simulink model "soc_dvbs2_fpga"  (R2025b)
settings: Solver=FixedStepDiscrete  StartTime=0.0  StopTime=0  RelTol=1e-3
InitFcn:
  | soc_dvbs2_init;
values from neighbouring files (symbols this model uses):
  Rsym = 4e6    (= 4000000)    [soc_dvbs2_init.m]
  soc_dvbs2_txPacketBits = [1 1 0 1 0 1 1 1 0 1 1 1 ... (2972 elements, 2972x1)]    [soc_dvbs2_txPacketBits.mat]
  syncWord = (dec2bin(hex2dec('AC')) - '0').'    [soc_dvbs2_init.m]
  txDataOut = txobj(frameBits(:))    [soc_dvbs2_init.m]
  txFiltCoeff = txobj.pTxFilterCoeff    [soc_dvbs2_init.m]
undefined symbols (not defined in the file or in its folder): Add, coefficientsLog, coefficientsSqrt1, coefficientsSqrt2, dataBits, designMultirateFIR, noisePow, NumBits1, NumBits2, seedsURNG1, seedsURNG2, Shift, Slope1, Slope2, soc_dvbs2_designFIRFilter, txDataOutS1, txDataOutS10, txDataOutS12, txDataOutS13, txDataOutS14, txDataOutS15, txDataOutS16, txDataOutS18, txDataOutS19, txDataOutS2, txDataOutS20, txDataOutS21, txDataOutS22, txDataOutS24, txDataOutS25, txDataOutS26, txDataOutS27, txDataOutS3, txDataOutS4, txDataOutS5, txDataOutS6, txDataOutS7, txDataOutS8, txDataOutS9
libraries: simulink x214, hdlsllib x211, dspsigops x22, dsphdlfiltering2 x8, dsphdlsigops2 x5, commseqgen3 x5, dsphdlmathfun2 x3, hwlogicconnlib x2, whdledac x2, commhdlcrc x2, whdlutilities x1, whdlmod x1
(part 10 of 12)

== system soc_dvbs2_fpga/DVBS2/DVBS2 TxRx/DVB-S2 HDL Receiver/Synchronizer and PL Header Decoder/Time Frequency and Coarse Phase Synchronizer/Fine Frequency Synchronizer/Modified L and R Algorithm/L and R Algorithm 18 point/Compute R(m) for 13 to 18/Compute R(m)_1 ==
  z : Inport
  zvalid : Inport  Port=2
  Add3 : Sum  Inputs=++|  OutDataTypeStr=Inherit: Inherit via back propagation
  Compare To Constant : simulink/Logic and Bit Operations/Compare To Constant  relop=>=  const=m  OutDataTypeStr=boolean
  Compare To Constant2 : simulink/Logic and Bit Operations/Compare To Constant  relop===  const=N - 1  OutDataTypeStr=boolean
  Complex Multiplier : Subsystem  VariantControl=Use 3 multipliers and 5 adders
      mask Display: disp(['Complex Multiplier' newline 'Latency = 8']);
  Data Type Duplicate : DataTypeDuplicate
  Data Type Conversion : DataTypeConversion  Commented=through  OutDataTypeStr=fixdt(1,28,17)  SaturateOnIntegerOverflow=off  RndMeth=Floor
  Delay : Delay  DelayLength=m
  Delay{1..2,7..9,11..12,14..15} (9 alike) : Delay  DelayLength=1
  Delay{3..6,10,13,16..26} (17 alike) : Delay
  Delay{27..30} (4 alike) : Delay  DelayLength=8
  Gain : Gain  Gain=MulDivFactor  ParamDataTypeStr=Inherit: Inherit from 'Gain'  OutDataTypeStr=Inherit: Same as input
  HDL Counter : hdlsllib/Sources/HDL Counter  CountType=Count limited  CountInit=0  CountStep=1  CountMax=N-1  CountFromType=Initial value  CountFrom=0  CountResetPort=off  CountLoadPort=off  CountEnbPort=on  CountDirPort=off  CountHitOutputPort=off  CountDataType=Unsigned  CountWordLen=nextpow2(N-1)  CountFracLen=0  CountSampTime=1
  Logical Operator : Logic  AllPortsSameDT=off  OutDataTypeStr=boolean
  Logical Operator1 : Logic  AllPortsSameDT=off  OutDataTypeStr=boolean
  Math Function : Math  Operator=conj
  Unit Delay Enabled Synchronous : hdlsllib/Discrete/Unit Delay Enabled Synchronous  InitialCondition=0.0  SampleTime=-1
  Unit Delay Enabled Resettable Synchronous : hdlsllib/Discrete/Unit Delay Enabled Resettable Synchronous  InitialCondition=0.0  SampleTime=-1
  Out1 : Outport
  wires:
  Data Type Conversion/1 -> Delay13/1
  Delay30/1 -> Delay20/1
  Delay29/1 -> Compare To Constant2/1
  Delay28/1 -> Compare To Constant/1
  Delay27/1 -> Delay17/1
  Delay13/1 -> Delay21/1
  Complex Multiplier/1(Out1) -> Data Type Conversion/1
  Delay26/1 -> Delay1/1
  Logical Operator/1 -> Delay25/1
  Delay24/1 -> Unit Delay Enabled Resettable Synchronous/2
  Delay23/1 -> Delay24/1
  Delay22/1 -> Add3/2, Data Type Duplicate/1
  Delay21/1 -> Gain/1
  Gain/1 -> Delay22/1
  Unit Delay Enabled Synchronous/1 -> Out1/1
  Delay20/1 -> Logical Operator/2
  Delay19/1 -> Logical Operator/1
  Delay18/1 -> Logical Operator1/2
  Delay17/1 -> Logical Operator1/1
  Delay16/1 -> Delay30/1
  Delay15/1 -> Delay16/1
  Delay12/1 -> Delay6/1
  Delay11/1 -> Delay5/1
  Delay10/1 -> Delay27/1
  Delay9/1 -> Delay10/1
  Delay8/1 -> Delay4/1
  Delay7/1 -> Delay3/1
  Delay6/1 -> Delay29/1
  Delay5/1 -> Delay28/1
  Delay4/1 -> Complex Multiplier/2(In2)
  Delay3/1 -> Complex Multiplier/1(In1)
  Delay2/1 -> Delay/1, Delay7/1
  Delay14/1 -> HDL Counter/1, Delay15/1, Delay9/1
  Math Function/1 -> Delay8/1
  z/1 -> Delay2/1
  Delay/1 -> Math Function/1
  Delay1/1 -> Unit Delay Enabled Resettable Synchronous/3, Unit Delay Enabled Synchronous/2
  Unit Delay Enabled Resettable Synchronous/1 -> Add3/1, Unit Delay Enabled Synchronous/1
  zvalid/1 -> Delay14/1
  Delay25/1 -> Delay26/1
  Compare To Constant2/1 -> Delay19/1
  Compare To Constant/1 -> Delay18/1
  HDL Counter/1 -> Delay12/1, Delay11/1
  Add3/1 -> Unit Delay Enabled Resettable Synchronous/1, Data Type Duplicate/2
  Logical Operator1/1 -> Delay23/1

== system soc_dvbs2_fpga/DVBS2/DVBS2 TxRx/DVB-S2 HDL Receiver/Synchronizer and PL Header Decoder/Time Frequency and Coarse Phase Synchronizer/Fine Frequency Synchronizer/Modified L and R Algorithm/L and R Algorithm 18 point/Compute R(m) for 13 to 18/Compute R(m)_2 ==
  z : Inport
  zvalid : Inport  Port=2
  Add3 : Sum  Inputs=++|  OutDataTypeStr=Inherit: Inherit via back propagation
  Compare To Constant : simulink/Logic and Bit Operations/Compare To Constant  relop=>=  const=m  OutDataTypeStr=boolean
  Compare To Constant2 : simulink/Logic and Bit Operations/Compare To Constant  relop===  const=N - 1  OutDataTypeStr=boolean
  Complex Multiplier : Subsystem  VariantControl=Use 3 multipliers and 5 adders
      mask Display: disp(['Complex Multiplier' newline 'Latency = 8']);
  Data Type Duplicate : DataTypeDuplicate
  Data Type Conversion : DataTypeConversion  Commented=through  OutDataTypeStr=fixdt(1,28,17)  SaturateOnIntegerOverflow=off  RndMeth=Floor
  Delay : Delay  DelayLength=m
  Delay{1..2,7..9,11..12,14..15} (9 alike) : Delay  DelayLength=1
  Delay{3..6,10,13,16..26} (17 alike) : Delay
  Delay{27..30} (4 alike) : Delay  DelayLength=8
  Gain : Gain  Gain=MulDivFactor  ParamDataTypeStr=Inherit: Inherit from 'Gain'  OutDataTypeStr=Inherit: Same as input
  HDL Counter : hdlsllib/Sources/HDL Counter  CountType=Count limited  CountInit=0  CountStep=1  CountMax=N-1  CountFromType=Initial value  CountFrom=0  CountResetPort=off  CountLoadPort=off  CountEnbPort=on  CountDirPort=off  CountHitOutputPort=off  CountDataType=Unsigned  CountWordLen=nextpow2(N-1)  CountFracLen=0  CountSampTime=1
  Logical Operator : Logic  AllPortsSameDT=off  OutDataTypeStr=boolean
  Logical Operator1 : Logic  AllPortsSameDT=off  OutDataTypeStr=boolean
  Math Function : Math  Operator=conj
  Unit Delay Enabled Synchronous : hdlsllib/Discrete/Unit Delay Enabled Synchronous  InitialCondition=0.0  SampleTime=-1
  Unit Delay Enabled Resettable Synchronous : hdlsllib/Discrete/Unit Delay Enabled Resettable Synchronous  InitialCondition=0.0  SampleTime=-1
  Out1 : Outport
  wires:
  Data Type Conversion/1 -> Delay13/1
  Logical Operator1/1 -> Delay23/1
  Add3/1 -> Data Type Duplicate/2, Unit Delay Enabled Resettable Synchronous/1
  HDL Counter/1 -> Delay11/1, Delay12/1
  Compare To Constant/1 -> Delay18/1
  Compare To Constant2/1 -> Delay19/1
  Delay25/1 -> Delay26/1
  zvalid/1 -> Delay14/1
  Unit Delay Enabled Resettable Synchronous/1 -> Unit Delay Enabled Synchronous/1, Add3/1
  Delay1/1 -> Unit Delay Enabled Synchronous/2, Unit Delay Enabled Resettable Synchronous/3
  Delay/1 -> Math Function/1
  z/1 -> Delay2/1
  Math Function/1 -> Delay8/1
  Delay14/1 -> Delay9/1, Delay15/1, HDL Counter/1
  Delay2/1 -> Delay7/1, Delay/1
  Delay3/1 -> Complex Multiplier/1(In1)
  Delay4/1 -> Complex Multiplier/2(In2)
  Delay5/1 -> Delay28/1
  Delay6/1 -> Delay29/1
  Delay7/1 -> Delay3/1
  Delay8/1 -> Delay4/1
  Delay9/1 -> Delay10/1
  Delay10/1 -> Delay27/1
  Delay11/1 -> Delay5/1
  Delay12/1 -> Delay6/1
  Delay15/1 -> Delay16/1
  Delay16/1 -> Delay30/1
  Delay17/1 -> Logical Operator1/1
  Delay18/1 -> Logical Operator1/2
  Delay19/1 -> Logical Operator/1
  Delay20/1 -> Logical Operator/2
  Unit Delay Enabled Synchronous/1 -> Out1/1
  Gain/1 -> Delay22/1
  Delay21/1 -> Gain/1
  Delay22/1 -> Data Type Duplicate/1, Add3/2
  Delay23/1 -> Delay24/1
  Delay24/1 -> Unit Delay Enabled Resettable Synchronous/2
  Logical Operator/1 -> Delay25/1
  Delay26/1 -> Delay1/1
  Complex Multiplier/1(Out1) -> Data Type Conversion/1
  Delay13/1 -> Delay21/1
  Delay27/1 -> Delay17/1
  Delay28/1 -> Compare To Constant/1
  Delay29/1 -> Compare To Constant2/1
  Delay30/1 -> Delay20/1

== system soc_dvbs2_fpga/DVBS2/DVBS2 TxRx/DVB-S2 HDL Receiver/Synchronizer and PL Header Decoder/Time Frequency and Coarse Phase Synchronizer/Fine Frequency Synchronizer/Modified L and R Algorithm/L and R Algorithm 18 point/Compute R(m) for 13 to 18/Compute R(m)_3 ==
  z : Inport
  zvalid : Inport  Port=2
  Add3 : Sum  Inputs=++|  OutDataTypeStr=Inherit: Inherit via back propagation
  Compare To Constant : simulink/Logic and Bit Operations/Compare To Constant  relop=>=  const=m  OutDataTypeStr=boolean
  Compare To Constant2 : simulink/Logic and Bit Operations/Compare To Constant  relop===  const=N - 1  OutDataTypeStr=boolean
  Complex Multiplier : Subsystem  VariantControl=Use 3 multipliers and 5 adders
      mask Display: disp(['Complex Multiplier' newline 'Latency = 8']);
  Data Type Duplicate : DataTypeDuplicate
  Data Type Conversion : DataTypeConversion  Commented=through  OutDataTypeStr=fixdt(1,28,17)  SaturateOnIntegerOverflow=off  RndMeth=Floor
  Delay : Delay  DelayLength=m
  Delay{1..2,7..9,11..12,14..15} (9 alike) : Delay  DelayLength=1
  Delay{3..6,10,13,16..26} (17 alike) : Delay
  Delay{27..30} (4 alike) : Delay  DelayLength=8
  Gain : Gain  Gain=MulDivFactor  ParamDataTypeStr=Inherit: Inherit from 'Gain'  OutDataTypeStr=Inherit: Same as input
  HDL Counter : hdlsllib/Sources/HDL Counter  CountType=Count limited  CountInit=0  CountStep=1  CountMax=N-1  CountFromType=Initial value  CountFrom=0  CountResetPort=off  CountLoadPort=off  CountEnbPort=on  CountDirPort=off  CountHitOutputPort=off  CountDataType=Unsigned  CountWordLen=nextpow2(N-1)  CountFracLen=0  CountSampTime=1
  Logical Operator : Logic  AllPortsSameDT=off  OutDataTypeStr=boolean
  Logical Operator1 : Logic  AllPortsSameDT=off  OutDataTypeStr=boolean
  Math Function : Math  Operator=conj
  Unit Delay Enabled Synchronous : hdlsllib/Discrete/Unit Delay Enabled Synchronous  InitialCondition=0.0  SampleTime=-1
  Unit Delay Enabled Resettable Synchronous : hdlsllib/Discrete/Unit Delay Enabled Resettable Synchronous  InitialCondition=0.0  SampleTime=-1
  Out1 : Outport
  wires:
  Data Type Conversion/1 -> Delay13/1
  Delay30/1 -> Delay20/1
  Delay29/1 -> Compare To Constant2/1
  Delay28/1 -> Compare To Constant/1
  Delay27/1 -> Delay17/1
  Delay13/1 -> Delay21/1
  Complex Multiplier/1(Out1) -> Data Type Conversion/1
  Delay26/1 -> Delay1/1
  Logical Operator/1 -> Delay25/1
  Delay24/1 -> Unit Delay Enabled Resettable Synchronous/2
  Delay23/1 -> Delay24/1
  Delay22/1 -> Add3/2, Data Type Duplicate/1
  Delay21/1 -> Gain/1
  Gain/1 -> Delay22/1
  Unit Delay Enabled Synchronous/1 -> Out1/1
  Delay20/1 -> Logical Operator/2
  Delay19/1 -> Logical Operator/1
  Delay18/1 -> Logical Operator1/2
  Delay17/1 -> Logical Operator1/1
  Delay16/1 -> Delay30/1
  Delay15/1 -> Delay16/1
  Delay12/1 -> Delay6/1
  Delay11/1 -> Delay5/1
  Delay10/1 -> Delay27/1
  Delay9/1 -> Delay10/1
  Delay8/1 -> Delay4/1
  Delay7/1 -> Delay3/1
  Delay6/1 -> Delay29/1
  Delay5/1 -> Delay28/1
  Delay4/1 -> Complex Multiplier/2(In2)
  Delay3/1 -> Complex Multiplier/1(In1)
  Delay2/1 -> Delay/1, Delay7/1
  Delay14/1 -> HDL Counter/1, Delay15/1, Delay9/1
  Math Function/1 -> Delay8/1
  z/1 -> Delay2/1
  Delay/1 -> Math Function/1
  Delay1/1 -> Unit Delay Enabled Resettable Synchronous/3, Unit Delay Enabled Synchronous/2
  Unit Delay Enabled Resettable Synchronous/1 -> Add3/1, Unit Delay Enabled Synchronous/1
  zvalid/1 -> Delay14/1
  Delay25/1 -> Delay26/1
  Compare To Constant2/1 -> Delay19/1
  Compare To Constant/1 -> Delay18/1
  HDL Counter/1 -> Delay12/1, Delay11/1
  Add3/1 -> Unit Delay Enabled Resettable Synchronous/1, Data Type Duplicate/2
  Logical Operator1/1 -> Delay23/1

== system soc_dvbs2_fpga/DVBS2/DVBS2 TxRx/DVB-S2 HDL Receiver/Synchronizer and PL Header Decoder/Time Frequency and Coarse Phase Synchronizer/Fine Frequency Synchronizer/Modified L and R Algorithm/L and R Algorithm 18 point/Compute R(m) for 13 to 18/Compute R(m)_4 ==
  z : Inport
  zvalid : Inport  Port=2
  Add3 : Sum  Inputs=++|  OutDataTypeStr=Inherit: Inherit via back propagation
  Compare To Constant : simulink/Logic and Bit Operations/Compare To Constant  relop=>=  const=m  OutDataTypeStr=boolean
  Compare To Constant2 : simulink/Logic and Bit Operations/Compare To Constant  relop===  const=N - 1  OutDataTypeStr=boolean
  Complex Multiplier : Subsystem  VariantControl=Use 3 multipliers and 5 adders
      mask Display: disp(['Complex Multiplier' newline 'Latency = 8']);
  Data Type Duplicate : DataTypeDuplicate
  Data Type Conversion : DataTypeConversion  Commented=through  OutDataTypeStr=fixdt(1,28,17)  SaturateOnIntegerOverflow=off  RndMeth=Floor
  Delay : Delay  DelayLength=m
  Delay{1..2,7..9,11..12,14..15} (9 alike) : Delay  DelayLength=1
  Delay{3..6,10,13,16..26} (17 alike) : Delay
  Delay{27..30} (4 alike) : Delay  DelayLength=8
  Gain : Gain  Gain=MulDivFactor  ParamDataTypeStr=Inherit: Inherit from 'Gain'  OutDataTypeStr=Inherit: Same as input
  HDL Counter : hdlsllib/Sources/HDL Counter  CountType=Count limited  CountInit=0  CountStep=1  CountMax=N-1  CountFromType=Initial value  CountFrom=0  CountResetPort=off  CountLoadPort=off  CountEnbPort=on  CountDirPort=off  CountHitOutputPort=off  CountDataType=Unsigned  CountWordLen=nextpow2(N-1)  CountFracLen=0  CountSampTime=1
  Logical Operator : Logic  AllPortsSameDT=off  OutDataTypeStr=boolean
  Logical Operator1 : Logic  AllPortsSameDT=off  OutDataTypeStr=boolean
  Math Function : Math  Operator=conj
  Unit Delay Enabled Synchronous : hdlsllib/Discrete/Unit Delay Enabled Synchronous  InitialCondition=0.0  SampleTime=-1
  Unit Delay Enabled Resettable Synchronous : hdlsllib/Discrete/Unit Delay Enabled Resettable Synchronous  InitialCondition=0.0  SampleTime=-1
  Out1 : Outport
  wires:
  Data Type Conversion/1 -> Delay13/1
  Logical Operator1/1 -> Delay23/1
  Add3/1 -> Data Type Duplicate/2, Unit Delay Enabled Resettable Synchronous/1
  HDL Counter/1 -> Delay11/1, Delay12/1
  Compare To Constant/1 -> Delay18/1
  Compare To Constant2/1 -> Delay19/1
  Delay25/1 -> Delay26/1
  zvalid/1 -> Delay14/1
  Unit Delay Enabled Resettable Synchronous/1 -> Unit Delay Enabled Synchronous/1, Add3/1
  Delay1/1 -> Unit Delay Enabled Synchronous/2, Unit Delay Enabled Resettable Synchronous/3
  Delay/1 -> Math Function/1
  z/1 -> Delay2/1
  Math Function/1 -> Delay8/1
  Delay14/1 -> Delay9/1, Delay15/1, HDL Counter/1
  Delay2/1 -> Delay7/1, Delay/1
  Delay3/1 -> Complex Multiplier/1(In1)
  Delay4/1 -> Complex Multiplier/2(In2)
  Delay5/1 -> Delay28/1
  Delay6/1 -> Delay29/1
  Delay7/1 -> Delay3/1
  Delay8/1 -> Delay4/1
  Delay9/1 -> Delay10/1
  Delay10/1 -> Delay27/1
  Delay11/1 -> Delay5/1
  Delay12/1 -> Delay6/1
  Delay15/1 -> Delay16/1
  Delay16/1 -> Delay30/1
  Delay17/1 -> Logical Operator1/1
  Delay18/1 -> Logical Operator1/2
  Delay19/1 -> Logical Operator/1
  Delay20/1 -> Logical Operator/2
  Unit Delay Enabled Synchronous/1 -> Out1/1
  Gain/1 -> Delay22/1
  Delay21/1 -> Gain/1
  Delay22/1 -> Data Type Duplicate/1, Add3/2
  Delay23/1 -> Delay24/1
  Delay24/1 -> Unit Delay Enabled Resettable Synchronous/2
  Logical Operator/1 -> Delay25/1
  Delay26/1 -> Delay1/1
  Complex Multiplier/1(Out1) -> Data Type Conversion/1
  Delay13/1 -> Delay21/1
  Delay27/1 -> Delay17/1
  Delay28/1 -> Compare To Constant/1
  Delay29/1 -> Compare To Constant2/1
  Delay30/1 -> Delay20/1

== system soc_dvbs2_fpga/DVBS2/DVBS2 TxRx/DVB-S2 HDL Receiver/Synchronizer and PL Header Decoder/Time Frequency and Coarse Phase Synchronizer/Fine Frequency Synchronizer/Modified L and R Algorithm/L and R Algorithm 18 point/Compute R(m) for 13 to 18/Compute R(m)_5 ==
  z : Inport
  zvalid : Inport  Port=2
  Add3 : Sum  Inputs=++|  OutDataTypeStr=Inherit: Inherit via back propagation
  Compare To Constant : simulink/Logic and Bit Operations/Compare To Constant  relop=>=  const=m  OutDataTypeStr=boolean
  Compare To Constant2 : simulink/Logic and Bit Operations/Compare To Constant  relop===  const=N - 1  OutDataTypeStr=boolean
  Complex Multiplier : Subsystem  VariantControl=Use 3 multipliers and 5 adders
      mask Display: disp(['Complex Multiplier' newline 'Latency = 8']);
  Data Type Duplicate : DataTypeDuplicate
  Data Type Conversion : DataTypeConversion  Commented=through  OutDataTypeStr=fixdt(1,28,17)  SaturateOnIntegerOverflow=off  RndMeth=Floor
  Delay : Delay  DelayLength=m
  Delay{1..2,7..9,11..12,14..15} (9 alike) : Delay  DelayLength=1
  Delay{3..6,10,13,16..26} (17 alike) : Delay
  Delay{27..30} (4 alike) : Delay  DelayLength=8
  Gain : Gain  Gain=MulDivFactor  ParamDataTypeStr=Inherit: Inherit from 'Gain'  OutDataTypeStr=Inherit: Same as input
  HDL Counter : hdlsllib/Sources/HDL Counter  CountType=Count limited  CountInit=0  CountStep=1  CountMax=N-1  CountFromType=Initial value  CountFrom=0  CountResetPort=off  CountLoadPort=off  CountEnbPort=on  CountDirPort=off  CountHitOutputPort=off  CountDataType=Unsigned  CountWordLen=nextpow2(N-1)  CountFracLen=0  CountSampTime=1
  Logical Operator : Logic  AllPortsSameDT=off  OutDataTypeStr=boolean
  Logical Operator1 : Logic  AllPortsSameDT=off  OutDataTypeStr=boolean
  Math Function : Math  Operator=conj
  Unit Delay Enabled Synchronous : hdlsllib/Discrete/Unit Delay Enabled Synchronous  InitialCondition=0.0  SampleTime=-1
  Unit Delay Enabled Resettable Synchronous : hdlsllib/Discrete/Unit Delay Enabled Resettable Synchronous  InitialCondition=0.0  SampleTime=-1
  Out1 : Outport
  wires:
  Data Type Conversion/1 -> Delay13/1
  Delay30/1 -> Delay20/1
  Delay29/1 -> Compare To Constant2/1
  Delay28/1 -> Compare To Constant/1
  Delay27/1 -> Delay17/1
  Delay13/1 -> Delay21/1
  Complex Multiplier/1(Out1) -> Data Type Conversion/1
  Delay26/1 -> Delay1/1
  Logical Operator/1 -> Delay25/1
  Delay24/1 -> Unit Delay Enabled Resettable Synchronous/2
  Delay23/1 -> Delay24/1
  Delay22/1 -> Add3/2, Data Type Duplicate/1
  Delay21/1 -> Gain/1
  Gain/1 -> Delay22/1
  Unit Delay Enabled Synchronous/1 -> Out1/1
  Delay20/1 -> Logical Operator/2
  Delay19/1 -> Logical Operator/1
  Delay18/1 -> Logical Operator1/2
  Delay17/1 -> Logical Operator1/1
  Delay16/1 -> Delay30/1
  Delay15/1 -> Delay16/1
  Delay12/1 -> Delay6/1
  Delay11/1 -> Delay5/1
  Delay10/1 -> Delay27/1
  Delay9/1 -> Delay10/1
  Delay8/1 -> Delay4/1
  Delay7/1 -> Delay3/1
  Delay6/1 -> Delay29/1
  Delay5/1 -> Delay28/1
  Delay4/1 -> Complex Multiplier/2(In2)
  Delay3/1 -> Complex Multiplier/1(In1)
  Delay2/1 -> Delay/1, Delay7/1
  Delay14/1 -> HDL Counter/1, Delay15/1, Delay9/1
  Math Function/1 -> Delay8/1
  z/1 -> Delay2/1
  Delay/1 -> Math Function/1
  Delay1/1 -> Unit Delay Enabled Resettable Synchronous/3, Unit Delay Enabled Synchronous/2
  Unit Delay Enabled Resettable Synchronous/1 -> Add3/1, Unit Delay Enabled Synchronous/1
  zvalid/1 -> Delay14/1
  Delay25/1 -> Delay26/1
  Compare To Constant2/1 -> Delay19/1
  Compare To Constant/1 -> Delay18/1
  HDL Counter/1 -> Delay12/1, Delay11/1
  Add3/1 -> Unit Delay Enabled Resettable Synchronous/1, Data Type Duplicate/2
  Logical Operator1/1 -> Delay23/1

== system soc_dvbs2_fpga/DVBS2/DVBS2 TxRx/DVB-S2 HDL Receiver/Synchronizer and PL Header Decoder/Time Frequency and Coarse Phase Synchronizer/Fine Frequency Synchronizer/Modified L and R Algorithm/L and R Algorithm 18 point/Compute R(m) for 13 to 18/Compute R(m)_6 ==
  z : Inport
  zvalid : Inport  Port=2
  Add3 : Sum  Inputs=++|  OutDataTypeStr=Inherit: Inherit via back propagation
  Compare To Constant : simulink/Logic and Bit Operations/Compare To Constant  relop=>=  const=m  OutDataTypeStr=boolean
  Compare To Constant2 : simulink/Logic and Bit Operations/Compare To Constant  relop===  const=N - 1  OutDataTypeStr=boolean
  Complex Multiplier : Subsystem  VariantControl=Use 3 multipliers and 5 adders
      mask Display: disp(['Complex Multiplier' newline 'Latency = 8']);
  Data Type Duplicate : DataTypeDuplicate
  Data Type Conversion : DataTypeConversion  Commented=through  OutDataTypeStr=fixdt(1,28,17)  SaturateOnIntegerOverflow=off  RndMeth=Floor
  Delay : Delay  DelayLength=m
  Delay{1..2,7..9,11..12,14..15} (9 alike) : Delay  DelayLength=1
  Delay{3..6,10,13,16..26} (17 alike) : Delay
  Delay{27..30} (4 alike) : Delay  DelayLength=8
  Gain : Gain  Gain=MulDivFactor  ParamDataTypeStr=Inherit: Inherit from 'Gain'  OutDataTypeStr=Inherit: Same as input
  HDL Counter : hdlsllib/Sources/HDL Counter  CountType=Count limited  CountInit=0  CountStep=1  CountMax=N-1  CountFromType=Initial value  CountFrom=0  CountResetPort=off  CountLoadPort=off  CountEnbPort=on  CountDirPort=off  CountHitOutputPort=off  CountDataType=Unsigned  CountWordLen=nextpow2(N-1)  CountFracLen=0  CountSampTime=1
  Logical Operator : Logic  AllPortsSameDT=off  OutDataTypeStr=boolean
  Logical Operator1 : Logic  AllPortsSameDT=off  OutDataTypeStr=boolean
  Math Function : Math  Operator=conj
  Unit Delay Enabled Synchronous : hdlsllib/Discrete/Unit Delay Enabled Synchronous  InitialCondition=0.0  SampleTime=-1
  Unit Delay Enabled Resettable Synchronous : hdlsllib/Discrete/Unit Delay Enabled Resettable Synchronous  InitialCondition=0.0  SampleTime=-1
  Out1 : Outport
  wires:
  Data Type Conversion/1 -> Delay13/1
  Logical Operator1/1 -> Delay23/1
  Add3/1 -> Data Type Duplicate/2, Unit Delay Enabled Resettable Synchronous/1
  HDL Counter/1 -> Delay11/1, Delay12/1
  Compare To Constant/1 -> Delay18/1
  Compare To Constant2/1 -> Delay19/1
  Delay25/1 -> Delay26/1
  zvalid/1 -> Delay14/1
  Unit Delay Enabled Resettable Synchronous/1 -> Unit Delay Enabled Synchronous/1, Add3/1
  Delay1/1 -> Unit Delay Enabled Synchronous/2, Unit Delay Enabled Resettable Synchronous/3
  Delay/1 -> Math Function/1
  z/1 -> Delay2/1
  Math Function/1 -> Delay8/1
  Delay14/1 -> Delay9/1, Delay15/1, HDL Counter/1
  Delay2/1 -> Delay7/1, Delay/1
  Delay3/1 -> Complex Multiplier/1(In1)
  Delay4/1 -> Complex Multiplier/2(In2)
  Delay5/1 -> Delay28/1
  Delay6/1 -> Delay29/1
  Delay7/1 -> Delay3/1
  Delay8/1 -> Delay4/1
  Delay9/1 -> Delay10/1
  Delay10/1 -> Delay27/1
  Delay11/1 -> Delay5/1
  Delay12/1 -> Delay6/1
  Delay15/1 -> Delay16/1
  Delay16/1 -> Delay30/1
  Delay17/1 -> Logical Operator1/1
  Delay18/1 -> Logical Operator1/2
  Delay19/1 -> Logical Operator/1
  Delay20/1 -> Logical Operator/2
  Unit Delay Enabled Synchronous/1 -> Out1/1
  Gain/1 -> Delay22/1
  Delay21/1 -> Gain/1
  Delay22/1 -> Data Type Duplicate/1, Add3/2
  Delay23/1 -> Delay24/1
  Delay24/1 -> Unit Delay Enabled Resettable Synchronous/2
  Logical Operator/1 -> Delay25/1
  Delay26/1 -> Delay1/1
  Complex Multiplier/1(Out1) -> Data Type Conversion/1
  Delay13/1 -> Delay21/1
  Delay27/1 -> Delay17/1
  Delay28/1 -> Compare To Constant/1
  Delay29/1 -> Compare To Constant2/1
  Delay30/1 -> Delay20/1

== system soc_dvbs2_fpga/DVBS2/DVBS2 TxRx/DVB-S2 HDL Receiver/Synchronizer and PL Header Decoder/Time Frequency and Coarse Phase Synchronizer/Fine Frequency Synchronizer/Modified L and R Algorithm/L and R Algorithm 18 point/Compute R(m) for 7 to 12/Compute R(m)_1 ==
  z : Inport
  zvalid : Inport  Port=2
  Add3 : Sum  Inputs=++|  OutDataTypeStr=Inherit: Inherit via back propagation
  Compare To Constant : simulink/Logic and Bit Operations/Compare To Constant  relop=>=  const=m  OutDataTypeStr=boolean
  Compare To Constant2 : simulink/Logic and Bit Operations/Compare To Constant  relop===  const=N - 1  OutDataTypeStr=boolean
  Complex Multiplier : Subsystem  VariantControl=Use 3 multipliers and 5 adders
      mask Display: disp(['Complex Multiplier' newline 'Latency = 8']);
  Data Type Duplicate : DataTypeDuplicate
  Data Type Conversion : DataTypeConversion  Commented=through  OutDataTypeStr=fixdt(1,28,17)  SaturateOnIntegerOverflow=off  RndMeth=Floor
  Delay : Delay  DelayLength=m
  Delay{1..2,7..9,11..12,14..15} (9 alike) : Delay  DelayLength=1
  Delay{3..6,10,13,16..26} (17 alike) : Delay
  Delay{27..30} (4 alike) : Delay  DelayLength=8
  Gain : Gain  Gain=MulDivFactor  ParamDataTypeStr=Inherit: Inherit from 'Gain'  OutDataTypeStr=Inherit: Same as input
  HDL Counter : hdlsllib/Sources/HDL Counter  CountType=Count limited  CountInit=0  CountStep=1  CountMax=N-1  CountFromType=Initial value  CountFrom=0  CountResetPort=off  CountLoadPort=off  CountEnbPort=on  CountDirPort=off  CountHitOutputPort=off  CountDataType=Unsigned  CountWordLen=nextpow2(N-1)  CountFracLen=0  CountSampTime=1
  Logical Operator : Logic  AllPortsSameDT=off  OutDataTypeStr=boolean
  Logical Operator1 : Logic  AllPortsSameDT=off  OutDataTypeStr=boolean
  Math Function : Math  Operator=conj
  Unit Delay Enabled Synchronous : hdlsllib/Discrete/Unit Delay Enabled Synchronous  InitialCondition=0.0  SampleTime=-1
  Unit Delay Enabled Resettable Synchronous : hdlsllib/Discrete/Unit Delay Enabled Resettable Synchronous  InitialCondition=0.0  SampleTime=-1
  Out1 : Outport
  wires:
  Logical Operator1/1 -> Delay23/1
  Add3/1 -> Data Type Duplicate/2, Unit Delay Enabled Resettable Synchronous/1
  HDL Counter/1 -> Delay11/1, Delay12/1
  Compare To Constant/1 -> Delay18/1
  Compare To Constant2/1 -> Delay19/1
  Delay25/1 -> Delay26/1
  zvalid/1 -> Delay14/1
  Unit Delay Enabled Resettable Synchronous/1 -> Unit Delay Enabled Synchronous/1, Add3/1
  Delay1/1 -> Unit Delay Enabled Synchronous/2, Unit Delay Enabled Resettable Synchronous/3
  Delay/1 -> Math Function/1
  z/1 -> Delay2/1
  Math Function/1 -> Delay8/1
  Delay14/1 -> Delay9/1, Delay15/1, HDL Counter/1
  Delay2/1 -> Delay7/1, Delay/1
  Delay3/1 -> Complex Multiplier/1(In1)
  Delay4/1 -> Complex Multiplier/2(In2)
  Delay5/1 -> Delay28/1
  Delay6/1 -> Delay29/1
  Delay7/1 -> Delay3/1
  Delay8/1 -> Delay4/1
  Delay9/1 -> Delay10/1
  Delay10/1 -> Delay27/1
  Delay11/1 -> Delay5/1
  Delay12/1 -> Delay6/1
  Delay15/1 -> Delay16/1
  Delay16/1 -> Delay30/1
  Delay17/1 -> Logical Operator1/1
  Delay18/1 -> Logical Operator1/2
  Delay19/1 -> Logical Operator/1
  Delay20/1 -> Logical Operator/2
  Unit Delay Enabled Synchronous/1 -> Out1/1
  Gain/1 -> Delay22/1
  Delay21/1 -> Gain/1
  Delay22/1 -> Data Type Duplicate/1, Add3/2
  Delay23/1 -> Delay24/1
  Delay24/1 -> Unit Delay Enabled Resettable Synchronous/2
  Logical Operator/1 -> Delay25/1
  Delay26/1 -> Delay1/1
  Complex Multiplier/1(Out1) -> Data Type Conversion/1
  Delay13/1 -> Delay21/1
  Delay27/1 -> Delay17/1
  Delay28/1 -> Compare To Constant/1
  Delay29/1 -> Compare To Constant2/1
  Delay30/1 -> Delay20/1
  Data Type Conversion/1 -> Delay13/1

== system soc_dvbs2_fpga/DVBS2/DVBS2 TxRx/DVB-S2 HDL Receiver/Synchronizer and PL Header Decoder/Time Frequency and Coarse Phase Synchronizer/Fine Frequency Synchronizer/Modified L and R Algorithm/L and R Algorithm 18 point/Compute R(m) for 7 to 12/Compute R(m)_2 ==
  z : Inport
  zvalid : Inport  Port=2
  Add3 : Sum  Inputs=++|  OutDataTypeStr=Inherit: Inherit via back propagation
  Compare To Constant : simulink/Logic and Bit Operations/Compare To Constant  relop=>=  const=m  OutDataTypeStr=boolean
  Compare To Constant2 : simulink/Logic and Bit Operations/Compare To Constant  relop===  const=N - 1  OutDataTypeStr=boolean
  Complex Multiplier : Subsystem  VariantControl=Use 3 multipliers and 5 adders
      mask Display: disp(['Complex Multiplier' newline 'Latency = 8']);
  Data Type Duplicate : DataTypeDuplicate
  Data Type Conversion : DataTypeConversion  Commented=through  OutDataTypeStr=fixdt(1,28,17)  SaturateOnIntegerOverflow=off  RndMeth=Floor
  Delay : Delay  DelayLength=m
  Delay{1..2,7..9,11..12,14..15} (9 alike) : Delay  DelayLength=1
  Delay{3..6,10,13,16..26} (17 alike) : Delay
  Delay{27..30} (4 alike) : Delay  DelayLength=8
  Gain : Gain  Gain=MulDivFactor  ParamDataTypeStr=Inherit: Inherit from 'Gain'  OutDataTypeStr=Inherit: Same as input
  HDL Counter : hdlsllib/Sources/HDL Counter  CountType=Count limited  CountInit=0  CountStep=1  CountMax=N-1  CountFromType=Initial value  CountFrom=0  CountResetPort=off  CountLoadPort=off  CountEnbPort=on  CountDirPort=off  CountHitOutputPort=off  CountDataType=Unsigned  CountWordLen=nextpow2(N-1)  CountFracLen=0  CountSampTime=1
  Logical Operator : Logic  AllPortsSameDT=off  OutDataTypeStr=boolean
  Logical Operator1 : Logic  AllPortsSameDT=off  OutDataTypeStr=boolean
  Math Function : Math  Operator=conj
  Unit Delay Enabled Synchronous : hdlsllib/Discrete/Unit Delay Enabled Synchronous  InitialCondition=0.0  SampleTime=-1
  Unit Delay Enabled Resettable Synchronous : hdlsllib/Discrete/Unit Delay Enabled Resettable Synchronous  InitialCondition=0.0  SampleTime=-1
  Out1 : Outport
  wires:
  Delay30/1 -> Delay20/1
  Delay29/1 -> Compare To Constant2/1
  Delay28/1 -> Compare To Constant/1
  Delay27/1 -> Delay17/1
  Delay13/1 -> Delay21/1
  Complex Multiplier/1(Out1) -> Data Type Conversion/1
  Delay26/1 -> Delay1/1
  Logical Operator/1 -> Delay25/1
  Delay24/1 -> Unit Delay Enabled Resettable Synchronous/2
  Delay23/1 -> Delay24/1
  Delay22/1 -> Add3/2, Data Type Duplicate/1
  Delay21/1 -> Gain/1
  Gain/1 -> Delay22/1
  Unit Delay Enabled Synchronous/1 -> Out1/1
  Delay20/1 -> Logical Operator/2
  Delay19/1 -> Logical Operator/1
  Delay18/1 -> Logical Operator1/2
  Delay17/1 -> Logical Operator1/1
  Delay16/1 -> Delay30/1
  Delay15/1 -> Delay16/1
  Delay12/1 -> Delay6/1
  Delay11/1 -> Delay5/1
  Delay10/1 -> Delay27/1
  Delay9/1 -> Delay10/1
  Delay8/1 -> Delay4/1
  Delay7/1 -> Delay3/1
  Delay6/1 -> Delay29/1
  Delay5/1 -> Delay28/1
  Delay4/1 -> Complex Multiplier/2(In2)
  Delay3/1 -> Complex Multiplier/1(In1)
  Delay2/1 -> Delay/1, Delay7/1
  Delay14/1 -> HDL Counter/1, Delay15/1, Delay9/1
  Math Function/1 -> Delay8/1
  z/1 -> Delay2/1
  Delay/1 -> Math Function/1
  Delay1/1 -> Unit Delay Enabled Resettable Synchronous/3, Unit Delay Enabled Synchronous/2
  Unit Delay Enabled Resettable Synchronous/1 -> Add3/1, Unit Delay Enabled Synchronous/1
  zvalid/1 -> Delay14/1
  Delay25/1 -> Delay26/1
  Compare To Constant2/1 -> Delay19/1
  Compare To Constant/1 -> Delay18/1
  HDL Counter/1 -> Delay12/1, Delay11/1
  Add3/1 -> Unit Delay Enabled Resettable Synchronous/1, Data Type Duplicate/2
  Logical Operator1/1 -> Delay23/1
  Data Type Conversion/1 -> Delay13/1

== system soc_dvbs2_fpga/DVBS2/DVBS2 TxRx/DVB-S2 HDL Receiver/Synchronizer and PL Header Decoder/Time Frequency and Coarse Phase Synchronizer/Fine Frequency Synchronizer/Modified L and R Algorithm/L and R Algorithm 18 point/Compute R(m) for 7 to 12/Compute R(m)_3 ==
  z : Inport
  zvalid : Inport  Port=2
  Add3 : Sum  Inputs=++|  OutDataTypeStr=Inherit: Inherit via back propagation
  Compare To Constant : simulink/Logic and Bit Operations/Compare To Constant  relop=>=  const=m  OutDataTypeStr=boolean
  Compare To Constant2 : simulink/Logic and Bit Operations/Compare To Constant  relop===  const=N - 1  OutDataTypeStr=boolean
  Complex Multiplier : Subsystem  VariantControl=Use 3 multipliers and 5 adders
      mask Display: disp(['Complex Multiplier' newline 'Latency = 8']);
  Data Type Duplicate : DataTypeDuplicate
  Data Type Conversion : DataTypeConversion  Commented=through  OutDataTypeStr=fixdt(1,28,17)  SaturateOnIntegerOverflow=off  RndMeth=Floor
  Delay : Delay  DelayLength=m
  Delay{1..2,7..9,11..12,14..15} (9 alike) : Delay  DelayLength=1
  Delay{3..6,10,13,16..26} (17 alike) : Delay
  Delay{27..30} (4 alike) : Delay  DelayLength=8
  Gain : Gain  Gain=MulDivFactor  ParamDataTypeStr=Inherit: Inherit from 'Gain'  OutDataTypeStr=Inherit: Same as input
  HDL Counter : hdlsllib/Sources/HDL Counter  CountType=Count limited  CountInit=0  CountStep=1  CountMax=N-1  CountFromType=Initial value  CountFrom=0  CountResetPort=off  CountLoadPort=off  CountEnbPort=on  CountDirPort=off  CountHitOutputPort=off  CountDataType=Unsigned  CountWordLen=nextpow2(N-1)  CountFracLen=0  CountSampTime=1
  Logical Operator : Logic  AllPortsSameDT=off  OutDataTypeStr=boolean
  Logical Operator1 : Logic  AllPortsSameDT=off  OutDataTypeStr=boolean
  Math Function : Math  Operator=conj
  Unit Delay Enabled Synchronous : hdlsllib/Discrete/Unit Delay Enabled Synchronous  InitialCondition=0.0  SampleTime=-1
  Unit Delay Enabled Resettable Synchronous : hdlsllib/Discrete/Unit Delay Enabled Resettable Synchronous  InitialCondition=0.0  SampleTime=-1
  Out1 : Outport
  wires:
  Logical Operator1/1 -> Delay23/1
  Add3/1 -> Data Type Duplicate/2, Unit Delay Enabled Resettable Synchronous/1
  HDL Counter/1 -> Delay11/1, Delay12/1
  Compare To Constant/1 -> Delay18/1
  Compare To Constant2/1 -> Delay19/1
  Delay25/1 -> Delay26/1
  zvalid/1 -> Delay14/1
  Unit Delay Enabled Resettable Synchronous/1 -> Unit Delay Enabled Synchronous/1, Add3/1
  Delay1/1 -> Unit Delay Enabled Synchronous/2, Unit Delay Enabled Resettable Synchronous/3
  Delay/1 -> Math Function/1
  z/1 -> Delay2/1
  Math Function/1 -> Delay8/1
  Delay14/1 -> Delay9/1, Delay15/1, HDL Counter/1
  Delay2/1 -> Delay7/1, Delay/1
  Delay3/1 -> Complex Multiplier/1(In1)
  Delay4/1 -> Complex Multiplier/2(In2)
  Delay5/1 -> Delay28/1
  Delay6/1 -> Delay29/1
  Delay7/1 -> Delay3/1
  Delay8/1 -> Delay4/1
  Delay9/1 -> Delay10/1
  Delay10/1 -> Delay27/1
  Delay11/1 -> Delay5/1
  Delay12/1 -> Delay6/1
  Delay15/1 -> Delay16/1
  Delay16/1 -> Delay30/1
  Delay17/1 -> Logical Operator1/1
  Delay18/1 -> Logical Operator1/2
  Delay19/1 -> Logical Operator/1
  Delay20/1 -> Logical Operator/2
  Unit Delay Enabled Synchronous/1 -> Out1/1
  Gain/1 -> Delay22/1
  Delay21/1 -> Gain/1
  Delay22/1 -> Data Type Duplicate/1, Add3/2
  Delay23/1 -> Delay24/1
  Delay24/1 -> Unit Delay Enabled Resettable Synchronous/2
  Logical Operator/1 -> Delay25/1
  Delay26/1 -> Delay1/1
  Complex Multiplier/1(Out1) -> Data Type Conversion/1
  Delay13/1 -> Delay21/1
  Delay27/1 -> Delay17/1
  Delay28/1 -> Compare To Constant/1
  Delay29/1 -> Compare To Constant2/1
  Delay30/1 -> Delay20/1
  Data Type Conversion/1 -> Delay13/1

== system soc_dvbs2_fpga/DVBS2/DVBS2 TxRx/DVB-S2 HDL Receiver/Synchronizer and PL Header Decoder/Time Frequency and Coarse Phase Synchronizer/Fine Frequency Synchronizer/Modified L and R Algorithm/L and R Algorithm 18 point/Compute R(m) for 7 to 12/Compute R(m)_4 ==
  z : Inport
  zvalid : Inport  Port=2
  Add3 : Sum  Inputs=++|  OutDataTypeStr=Inherit: Inherit via back propagation
  Compare To Constant : simulink/Logic and Bit Operations/Compare To Constant  relop=>=  const=m  OutDataTypeStr=boolean
  Compare To Constant2 : simulink/Logic and Bit Operations/Compare To Constant  relop===  const=N - 1  OutDataTypeStr=boolean
  Complex Multiplier : Subsystem  VariantControl=Use 3 multipliers and 5 adders
      mask Display: disp(['Complex Multiplier' newline 'Latency = 8']);
  Data Type Duplicate : DataTypeDuplicate
  Data Type Conversion : DataTypeConversion  Commented=through  OutDataTypeStr=fixdt(1,28,17)  SaturateOnIntegerOverflow=off  RndMeth=Floor
  Delay : Delay  DelayLength=m
  Delay{1..2,7..9,11..12,14..15} (9 alike) : Delay  DelayLength=1
  Delay{3..6,10,13,16..26} (17 alike) : Delay
  Delay{27..30} (4 alike) : Delay  DelayLength=8
  Gain : Gain  Gain=MulDivFactor  ParamDataTypeStr=Inherit: Inherit from 'Gain'  OutDataTypeStr=Inherit: Same as input
  HDL Counter : hdlsllib/Sources/HDL Counter  CountType=Count limited  CountInit=0  CountStep=1  CountMax=N-1  CountFromType=Initial value  CountFrom=0  CountResetPort=off  CountLoadPort=off  CountEnbPort=on  CountDirPort=off  CountHitOutputPort=off  CountDataType=Unsigned  CountWordLen=nextpow2(N-1)  CountFracLen=0  CountSampTime=1
  Logical Operator : Logic  AllPortsSameDT=off  OutDataTypeStr=boolean
  Logical Operator1 : Logic  AllPortsSameDT=off  OutDataTypeStr=boolean
  Math Function : Math  Operator=conj
  Unit Delay Enabled Synchronous : hdlsllib/Discrete/Unit Delay Enabled Synchronous  InitialCondition=0.0  SampleTime=-1
  Unit Delay Enabled Resettable Synchronous : hdlsllib/Discrete/Unit Delay Enabled Resettable Synchronous  InitialCondition=0.0  SampleTime=-1
  Out1 : Outport
  wires:
  Delay30/1 -> Delay20/1
  Delay29/1 -> Compare To Constant2/1
  Delay28/1 -> Compare To Constant/1
  Delay27/1 -> Delay17/1
  Delay13/1 -> Delay21/1
  Complex Multiplier/1(Out1) -> Data Type Conversion/1
  Delay26/1 -> Delay1/1
  Logical Operator/1 -> Delay25/1
  Delay24/1 -> Unit Delay Enabled Resettable Synchronous/2
  Delay23/1 -> Delay24/1
  Delay22/1 -> Add3/2, Data Type Duplicate/1
  Delay21/1 -> Gain/1
  Gain/1 -> Delay22/1
  Unit Delay Enabled Synchronous/1 -> Out1/1
  Delay20/1 -> Logical Operator/2
  Delay19/1 -> Logical Operator/1
  Delay18/1 -> Logical Operator1/2
  Delay17/1 -> Logical Operator1/1
  Delay16/1 -> Delay30/1
  Delay15/1 -> Delay16/1
  Delay12/1 -> Delay6/1
  Delay11/1 -> Delay5/1
  Delay10/1 -> Delay27/1
  Delay9/1 -> Delay10/1
  Delay8/1 -> Delay4/1
  Delay7/1 -> Delay3/1
  Delay6/1 -> Delay29/1
  Delay5/1 -> Delay28/1
  Delay4/1 -> Complex Multiplier/2(In2)
  Delay3/1 -> Complex Multiplier/1(In1)
  Delay2/1 -> Delay/1, Delay7/1
  Delay14/1 -> HDL Counter/1, Delay15/1, Delay9/1
  Math Function/1 -> Delay8/1
  z/1 -> Delay2/1
  Delay/1 -> Math Function/1
  Delay1/1 -> Unit Delay Enabled Resettable Synchronous/3, Unit Delay Enabled Synchronous/2
  Unit Delay Enabled Resettable Synchronous/1 -> Add3/1, Unit Delay Enabled Synchronous/1
  zvalid/1 -> Delay14/1
  Delay25/1 -> Delay26/1
  Compare To Constant2/1 -> Delay19/1
  Compare To Constant/1 -> Delay18/1
  HDL Counter/1 -> Delay12/1, Delay11/1
  Add3/1 -> Unit Delay Enabled Resettable Synchronous/1, Data Type Duplicate/2
  Logical Operator1/1 -> Delay23/1
  Data Type Conversion/1 -> Delay13/1

== system soc_dvbs2_fpga/DVBS2/DVBS2 TxRx/DVB-S2 HDL Receiver/Synchronizer and PL Header Decoder/Time Frequency and Coarse Phase Synchronizer/Fine Frequency Synchronizer/Modified L and R Algorithm/L and R Algorithm 18 point/Compute R(m) for 7 to 12/Compute R(m)_5 ==
  z : Inport
  zvalid : Inport  Port=2
  Add3 : Sum  Inputs=++|  OutDataTypeStr=Inherit: Inherit via back propagation
  Compare To Constant : simulink/Logic and Bit Operations/Compare To Constant  relop=>=  const=m  OutDataTypeStr=boolean
  Compare To Constant2 : simulink/Logic and Bit Operations/Compare To Constant  relop===  const=N - 1  OutDataTypeStr=boolean
  Complex Multiplier : Subsystem  VariantControl=Use 3 multipliers and 5 adders
      mask Display: disp(['Complex Multiplier' newline 'Latency = 8']);
  Data Type Duplicate : DataTypeDuplicate
  Data Type Conversion : DataTypeConversion  Commented=through  OutDataTypeStr=fixdt(1,28,17)  SaturateOnIntegerOverflow=off  RndMeth=Floor
  Delay : Delay  DelayLength=m
  Delay{1..2,7..9,11..12,14..15} (9 alike) : Delay  DelayLength=1
  Delay{3..6,10,13,16..26} (17 alike) : Delay
  Delay{27..30} (4 alike) : Delay  DelayLength=8
  Gain : Gain  Gain=MulDivFactor  ParamDataTypeStr=Inherit: Inherit from 'Gain'  OutDataTypeStr=Inherit: Same as input
  HDL Counter : hdlsllib/Sources/HDL Counter  CountType=Count limited  CountInit=0  CountStep=1  CountMax=N-1  CountFromType=Initial value  CountFrom=0  CountResetPort=off  CountLoadPort=off  CountEnbPort=on  CountDirPort=off  CountHitOutputPort=off  CountDataType=Unsigned  CountWordLen=nextpow2(N-1)  CountFracLen=0  CountSampTime=1
  Logical Operator : Logic  AllPortsSameDT=off  OutDataTypeStr=boolean
  Logical Operator1 : Logic  AllPortsSameDT=off  OutDataTypeStr=boolean
  Math Function : Math  Operator=conj
  Unit Delay Enabled Synchronous : hdlsllib/Discrete/Unit Delay Enabled Synchronous  InitialCondition=0.0  SampleTime=-1
  Unit Delay Enabled Resettable Synchronous : hdlsllib/Discrete/Unit Delay Enabled Resettable Synchronous  InitialCondition=0.0  SampleTime=-1
  Out1 : Outport
  wires:
  Logical Operator1/1 -> Delay23/1
  Add3/1 -> Data Type Duplicate/2, Unit Delay Enabled Resettable Synchronous/1
  HDL Counter/1 -> Delay11/1, Delay12/1
  Compare To Constant/1 -> Delay18/1
  Compare To Constant2/1 -> Delay19/1
  Delay25/1 -> Delay26/1
  zvalid/1 -> Delay14/1
  Unit Delay Enabled Resettable Synchronous/1 -> Unit Delay Enabled Synchronous/1, Add3/1
  Delay1/1 -> Unit Delay Enabled Synchronous/2, Unit Delay Enabled Resettable Synchronous/3
  Delay/1 -> Math Function/1
  z/1 -> Delay2/1
  Math Function/1 -> Delay8/1
  Delay14/1 -> Delay9/1, Delay15/1, HDL Counter/1
  Delay2/1 -> Delay7/1, Delay/1
  Delay3/1 -> Complex Multiplier/1(In1)
  Delay4/1 -> Complex Multiplier/2(In2)
  Delay5/1 -> Delay28/1
  Delay6/1 -> Delay29/1
  Delay7/1 -> Delay3/1
  Delay8/1 -> Delay4/1
  Delay9/1 -> Delay10/1
  Delay10/1 -> Delay27/1
  Delay11/1 -> Delay5/1
  Delay12/1 -> Delay6/1
  Delay15/1 -> Delay16/1
  Delay16/1 -> Delay30/1
  Delay17/1 -> Logical Operator1/1
  Delay18/1 -> Logical Operator1/2
  Delay19/1 -> Logical Operator/1
  Delay20/1 -> Logical Operator/2
  Unit Delay Enabled Synchronous/1 -> Out1/1
  Gain/1 -> Delay22/1
  Delay21/1 -> Gain/1
  Delay22/1 -> Data Type Duplicate/1, Add3/2
  Delay23/1 -> Delay24/1
  Delay24/1 -> Unit Delay Enabled Resettable Synchronous/2
  Logical Operator/1 -> Delay25/1
  Delay26/1 -> Delay1/1
  Complex Multiplier/1(Out1) -> Data Type Conversion/1
  Delay13/1 -> Delay21/1
  Delay27/1 -> Delay17/1
  Delay28/1 -> Compare To Constant/1
  Delay29/1 -> Compare To Constant2/1
  Delay30/1 -> Delay20/1
  Data Type Conversion/1 -> Delay13/1

== system soc_dvbs2_fpga/DVBS2/DVBS2 TxRx/DVB-S2 HDL Receiver/Synchronizer and PL Header Decoder/Time Frequency and Coarse Phase Synchronizer/Fine Frequency Synchronizer/Modified L and R Algorithm/L and R Algorithm 18 point/Compute R(m) for 7 to 12/Compute R(m)_6 ==
  z : Inport
  zvalid : Inport  Port=2
  Add3 : Sum  Inputs=++|  OutDataTypeStr=Inherit: Inherit via back propagation
  Compare To Constant : simulink/Logic and Bit Operations/Compare To Constant  relop=>=  const=m  OutDataTypeStr=boolean
  Compare To Constant2 : simulink/Logic and Bit Operations/Compare To Constant  relop===  const=N - 1  OutDataTypeStr=boolean
  Complex Multiplier : Subsystem  VariantControl=Use 3 multipliers and 5 adders
      mask Display: disp(['Complex Multiplier' newline 'Latency = 8']);
  Data Type Duplicate : DataTypeDuplicate
  Data Type Conversion : DataTypeConversion  Commented=through  OutDataTypeStr=fixdt(1,28,17)  SaturateOnIntegerOverflow=off  RndMeth=Floor
  Delay : Delay  DelayLength=m
  Delay{1..2,7..9,11..12,14..15} (9 alike) : Delay  DelayLength=1
  Delay{3..6,10,13,16..26} (17 alike) : Delay
  Delay{27..30} (4 alike) : Delay  DelayLength=8
  Gain : Gain  Gain=MulDivFactor  ParamDataTypeStr=Inherit: Inherit from 'Gain'  OutDataTypeStr=Inherit: Same as input
  HDL Counter : hdlsllib/Sources/HDL Counter  CountType=Count limited  CountInit=0  CountStep=1  CountMax=N-1  CountFromType=Initial value  CountFrom=0  CountResetPort=off  CountLoadPort=off  CountEnbPort=on  CountDirPort=off  CountHitOutputPort=off  CountDataType=Unsigned  CountWordLen=nextpow2(N-1)  CountFracLen=0  CountSampTime=1
  Logical Operator : Logic  AllPortsSameDT=off  OutDataTypeStr=boolean
  Logical Operator1 : Logic  AllPortsSameDT=off  OutDataTypeStr=boolean
  Math Function : Math  Operator=conj
  Unit Delay Enabled Synchronous : hdlsllib/Discrete/Unit Delay Enabled Synchronous  InitialCondition=0.0  SampleTime=-1
  Unit Delay Enabled Resettable Synchronous : hdlsllib/Discrete/Unit Delay Enabled Resettable Synchronous  InitialCondition=0.0  SampleTime=-1
  Out1 : Outport
  wires:
  Delay30/1 -> Delay20/1
  Delay29/1 -> Compare To Constant2/1
  Delay28/1 -> Compare To Constant/1
  Delay27/1 -> Delay17/1
  Delay13/1 -> Delay21/1
  Complex Multiplier/1(Out1) -> Data Type Conversion/1
  Delay26/1 -> Delay1/1
  Logical Operator/1 -> Delay25/1
  Delay24/1 -> Unit Delay Enabled Resettable Synchronous/2
  Delay23/1 -> Delay24/1
  Delay22/1 -> Add3/2, Data Type Duplicate/1
  Delay21/1 -> Gain/1
  Gain/1 -> Delay22/1
  Unit Delay Enabled Synchronous/1 -> Out1/1
  Delay20/1 -> Logical Operator/2
  Delay19/1 -> Logical Operator/1
  Delay18/1 -> Logical Operator1/2
  Delay17/1 -> Logical Operator1/1
  Delay16/1 -> Delay30/1
  Delay15/1 -> Delay16/1
  Delay12/1 -> Delay6/1
  Delay11/1 -> Delay5/1
  Delay10/1 -> Delay27/1
  Delay9/1 -> Delay10/1
  Delay8/1 -> Delay4/1
  Delay7/1 -> Delay3/1
  Delay6/1 -> Delay29/1
  Delay5/1 -> Delay28/1
  Delay4/1 -> Complex Multiplier/2(In2)
  Delay3/1 -> Complex Multiplier/1(In1)
  Delay2/1 -> Delay/1, Delay7/1
  Delay14/1 -> HDL Counter/1, Delay15/1, Delay9/1
  Math Function/1 -> Delay8/1
  z/1 -> Delay2/1
  Delay/1 -> Math Function/1
  Delay1/1 -> Unit Delay Enabled Resettable Synchronous/3, Unit Delay Enabled Synchronous/2
  Unit Delay Enabled Resettable Synchronous/1 -> Add3/1, Unit Delay Enabled Synchronous/1
  zvalid/1 -> Delay14/1
  Delay25/1 -> Delay26/1
  Compare To Constant2/1 -> Delay19/1
  Compare To Constant/1 -> Delay18/1
  HDL Counter/1 -> Delay12/1, Delay11/1
  Add3/1 -> Unit Delay Enabled Resettable Synchronous/1, Data Type Duplicate/2
  Logical Operator1/1 -> Delay23/1
  Data Type Conversion/1 -> Delay13/1

== system soc_dvbs2_fpga/DVBS2/DVBS2 TxRx/DVB-S2 HDL Receiver/Synchronizer and PL Header Decoder/Time Frequency and Coarse Phase Synchronizer/Time and Coarse Frequency Synchronizer/PL Data Descrambler and Pilot Valid Indicator/PL Data Descrambler/PL Scrambler Gold Sequence Generator/Subsystem ==
  note: The initial output of these outports are set to 0 as this is an enabled subsystem
  reset : Inport
  Enable : EnablePort
  X PN Generator M_n : commseqgen3/PN Sequence Generator  poly='z^18+z^7+1'  ini_sta=[zeros(1,17) 1]  outBitMaskSource=Dialog parameter  shift=n  outVarSiz=off  maxOutSizeMode=Dialog parameter  maxOutSize=[10 1]  Ts=-1  sampPerFrame=1  reset=on  bitPackedOutputs=off  outDataType=boolean  numPackedBits=8  bitPackDataSigned=off  bitPackedOutDType=double
  X PN Generator M_nplus131072 : commseqgen3/PN Sequence Generator  poly='z^18+z^7+1'  ini_sta=[zeros(1,17) 1]  outBitMaskSource=Dialog parameter  shift=n+131072  outVarSiz=off  maxOutSizeMode=Dialog parameter  maxOutSize=[10 1]  Ts=-1  sampPerFrame=1  reset=on  bitPackedOutputs=off  outDataType=boolean  numPackedBits=8  bitPackDataSigned=off  bitPackedOutDType=double
  Y PN Generator M_0 : commseqgen3/PN Sequence Generator  poly='z^18 + z^10 + z^7 + z^5 + 1'  ini_sta=ones(1,18)  outBitMaskSource=Dialog parameter  shift=0  outVarSiz=off  maxOutSizeMode=Dialog parameter  maxOutSize=[10 1]  Ts=-1  sampPerFrame=1  reset=on  bitPackedOutputs=off  outDataType=boolean  numPackedBits=8  bitPackDataSigned=off  bitPackedOutDType=double
  Y PN Generator M_131072 : commseqgen3/PN Sequence Generator  poly='z^18 + z^10 + z^7 + z^5 + 1'  ini_sta=ones(1,18)  outBitMaskSource=Dialog parameter  shift=131072  outVarSiz=off  maxOutSizeMode=Dialog parameter  maxOutSize=[10 1]  Ts=-1  sampPerFrame=1  reset=on  bitPackedOutputs=off  outDataType=boolean  numPackedBits=8  bitPackDataSigned=off  bitPackedOutDType=double
  xMnp131072 : Outport  InitialOutput=0
  yM131072 : Outport  Port=2  InitialOutput=0
  xMn : Outport  Port=3  InitialOutput=0
  yM0 : Outport  Port=4  InitialOutput=0
  wires:
  Y PN Generator M_131072/1 -> yM131072/1
  X PN Generator M_n/1 -> xMn/1
  reset/1 -> Y PN Generator M_131072/1, X PN Generator M_n/1, Y PN Generator M_0/1, X PN Generator M_nplus131072/1
  Y PN Generator M_0/1 -> yM0/1
  X PN Generator M_nplus131072/1 -> xMnp131072/1
